simulink model "PID_Controller"  (R2014a)
settings: Solver=ode45  StartTime=0.0  StopTime=10.0  RelTol=1e-3
libraries: simulink x1
settings Model: Creator=mamta  LastModifiedBy=mamta

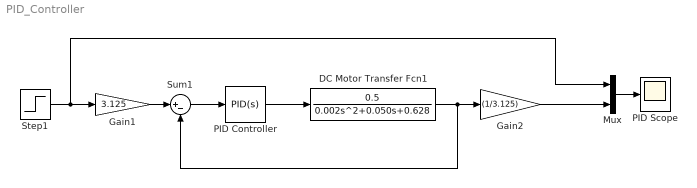
== system PID_Controller ==
  DC Motor Transfer Fcn1 : TransferFcn  Numerator=[0.5]  Denominator=[0.002 0.050 0.628]
  Gain1 : Gain  Gain=3.125
  Gain2 : Gain  Gain=(1/3.125)
  Mux : Mux  Inputs=2
  PID Controller : simulink/Continuous/PID Controller  Controller=PID  TimeDomain=Continuous-time  SampleTime=1  IntegratorMethod=Forward Euler  FilterMethod=Forward Euler  Form=Parallel  P=11.2553274186345  I=55.2865830133075  D=0.0841202764436933  N=83.310900837003  InitialConditionSource=internal  InitialConditionForIntegrator=0  InitialConditionForFilter=0  ExternalReset=none  LimitOutput=off  UpperSaturationLimit=inf  LowerSaturationLimit=-inf  LinearizeAsGain=on  AntiWindupMode=none  Kb=1  TrackingMode=off  Kt=1  PParamMin=[]  PParamMax=[]  IParamMin=[]  IParamMax=[]  DParamMin=[]  DParamMax=[]  NParamMin=[]  NParamMax=[]  KbParamMin=[]  KbParamMax=[]  KtParamMin=[]  KtParamMax=[]  POutMin=[]  POutMax=[]  IOutMin=[]  IOutMax=[]  DOutMin=[]  DOutMax=[]  NOutMin=[]  NOutMax=[]  KbOutMin=[]  KbOutMax=[]  KtOutMin=[]  KtOutMax=[]  IntegratorOutMin=[]  IntegratorOutMax=[]  FilterOutMin=[]  FilterOutMax=[]  SumOutMin=[]  SumOutMax=[]  SumI1OutMin=[]  SumI1OutMax=[]  SumI2OutMin=[]  SumI2OutMax=[]  SumI3OutMin=[]  SumI3OutMax=[]  SumDOutMin=[]  SumDOutMax=[]  SaturationOutMin=[]  SaturationOutMax=[]  IntegratorContinuousStateAttributes=''  IntegratorStateMustResolveToSignalObject=off  IntegratorRTWStateStorageClass=Auto  FilterContinuousStateAttributes=''  FilterStateMustResolveToSignalObject=off  FilterRTWStateStorageClass=Auto
  PID Scope : Scope
      settings: YMin=0.99935  YMax=1
  Step1 : Step  Time=0  SampleTime=0
  Sum1 : Sum  Inputs=|+-
  wires:
  Sum1/1 -> PID Controller/1
  PID Controller/1 -> DC Motor Transfer Fcn1/1
  DC Motor Transfer Fcn1/1 -> Sum1/2, Gain2/1
  Gain1/1 -> Sum1/1
  Gain2/1 -> Mux/2
  Step1/1 -> Mux/1, Gain1/1
  Mux/1 -> PID Scope/1
